simulink model "RequirementTable_testing"  (R2022b)
settings: Solver=FixedStepAuto  StartTime=0.0  StopTime=10.0  FixedStep=1e-3  RelTol=1e-3  EnableMultiTasking=on
undefined symbols (not defined in the file): D0, D1, D10, D11, D12, D13, D2, D3, D4, D5, D6, D7, D8, D9, PTA0, PTA1, PTA2, PTB23, PTB9, PTC16, PTC17, PTC2, PTC3, PTC4, PTD0, PTD1, PTD2, PTD3
libraries: frdmk64flib x18, dspstat3 x1
settings Model: SimulationMode=external  ExtModeTrigDuration=5  Creator=sarahalabdulrazzak  LastModifiedBy=coler
settings SolverCC: AlgebraicLoopSolver=TrustRegion
settings OptimizationCC: EnhancedBackFolding=on  PassReuseOutputArgsAs=Individual arguments  ZeroExternalMemoryAtStartup=off  ZeroInternalMemoryAtStartup=off  MaxStackSize=64  OptimizeBlockOrder=speed  DifferentSizesBufferReuse=on  OptimizationCustomize=off  EfficientTunableParamExpr=on
settings DebuggingCC: ParameterTunabilityLossMsg=error  UnconnectedInputMsg=warning  UnconnectedOutputMsg=warning  UnconnectedLineMsg=warning  SFMachineParentedDataDiag=warning
settings HardwareCC: ProdBitPerPointer=32  ProdBitPerSizeT=32  ProdBitPerPtrDiffT=32  ProdLargestAtomicInteger=Long  ProdLargestAtomicFloat=Double  ProdWordSize=32  ProdHWDeviceType=ARM Compatible->ARM Cortex
settings ModelReferenceCC: EnableRefExpFcnMdlSchedulingChecks=on
settings SFSimCC: MATLABDynamicMemAlloc=off
settings RTWCC: Description=Embedded Coder  SystemTargetFile=ert.tlc  HardwareBoard=NXP FRDM-K64F  TLCOptions="-aInlineSetEventsForThisBaseRateFcn=TLC_FALSE -aSuppressMultiTaskScheduler=TLC_FALSE  -aRateBasedStepFcn=0"  TemplateMakefile=ert_default_tmf  Toolchain=GNU Tools for ARM Embedded Processors
settings CodeAppCC: ForceParamTrailComments=on  IgnoreCustomStorageClasses=off  OperatorAnnotations=on  SimulinkDataObjDesc=on  SFDataObjDesc=on  InsertBlockDesc=on
settings ERTTargetCC: ExtMode=on  ExtModeTransport=4  ExtModeMexFile=sendToCommService  ExtModeMexArgs='RA_Modes' 0

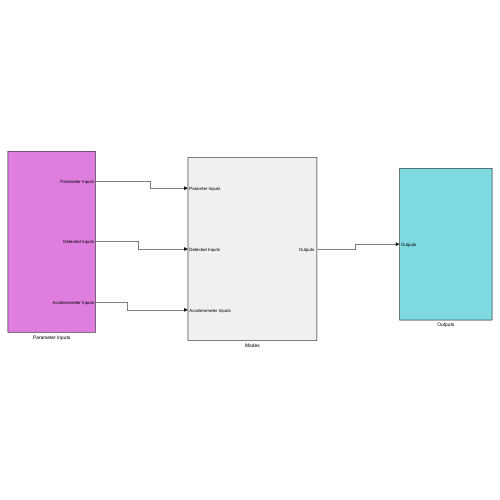
[thumbnail: Simulink's stored preview of the top-level diagram]
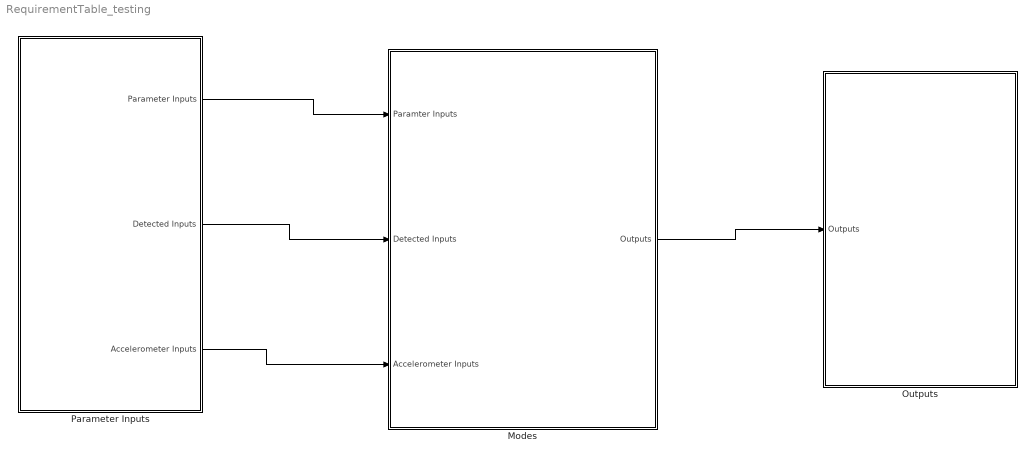
== system RequirementTable_testing ==
  Modes : Subsystem
  Outputs : Subsystem
  Parameter Inputs : Subsystem
  wires:
  Parameter Inputs/1(Parameter Inputs) -> Modes/1(Paramter Inputs)
  Parameter Inputs/2(Detected Inputs) -> Modes/2(Detected Inputs)
  Modes/1("Outputs ") -> Outputs/1("Outputs ")
  Parameter Inputs/3(Accelerometer Inputs) -> Modes/3(Accelerometer Inputs)

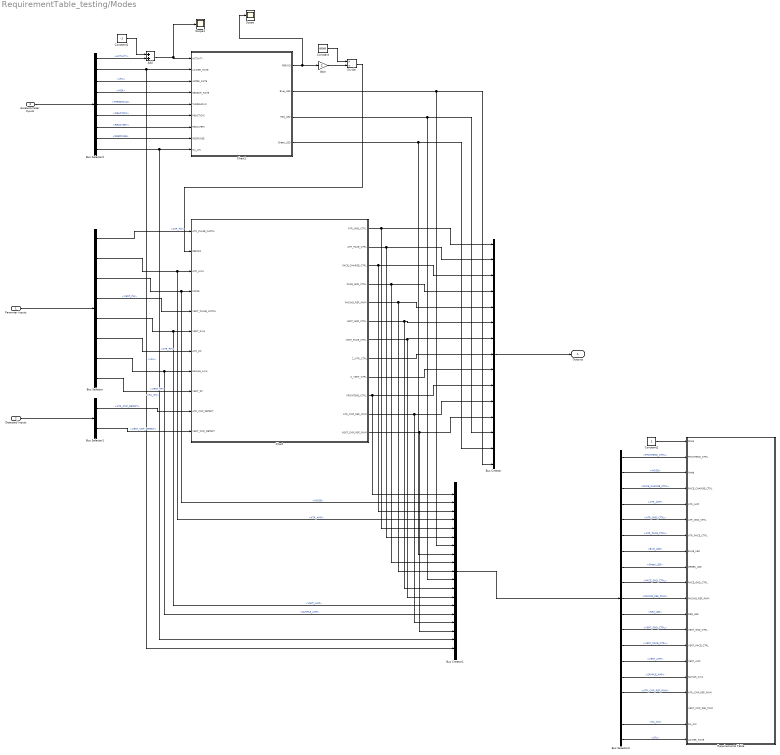
== system RequirementTable_testing/Modes ==
  Paramter Inputs : Inport
  Detected Inputs : Inport  Port=2
  Accelerometer Inputs : Inport  Port=3
  Add : Sum
  Bus Creator : BusCreator  Inputs=15
  Bus Creator1 : BusCreator  Inputs=19
  Bus Selector : BusSelector  OutputSignals=ATR_PW,ATR_AMP,MODE,VENT_PW,VENT_AMP,ATR_RP,SAMPLE_AMP,VENT_RP
  Bus Selector1 : BusSelector  OutputSignals=ATR_CMP_DETECT,VENT_CMP_DETECT
  Bus Selector2 : BusSelector  OutputSignals=ACTIVITY,LRL,URL,MSR,THRESHOLD,REACTION,RECOVERY,RESPONSE,RA_ON
  Bus Selector3 : BusSelector  OutputSignals=FRONTEND_CTRL,MODE,PACE_CHARGE_CTRL,ATR_AMP,ATR_GND_CTRL,ATR_PACE_CTRL,Blue_LED,Green_LED,PACE_GND_CTRL,PACING_REF_PWM,Red_LED,VENT_GND_CTRL,VENT_PACE_CTRL,VENT_AMP,SAMPLE_AMP,ATR_CMP_REF_PWM,VENT_CMP_REF_PWM,RA_ON,LRL
  Chart : Stateflow chart  TreatAsAtomicUnit=on
  Chart1 : Stateflow chart  TreatAsAtomicUnit=on
  Constant : Constant  Value=60000
  Constant1 : Constant  Value=-1
  Constant2 : Constant
  Divide : Product  Inputs=*/
  Gain : Gain  Gain=2
  Requirements Table : Requirements Table  TreatAsAtomicUnit=on
  Scope : Scope
  Scope1 : Scope
  "Outputs " : Outport
  wires:
  Paramter Inputs/1 -> Bus Selector/1
  Detected Inputs/1 -> Bus Selector1/1
  Bus Selector/1 -> Chart/1(ATR_PULSE_WIDTH)  "<ATR_PW>"
  Chart/1(ATR_GND_CTRL) -> Bus Creator1/5, Bus Creator/1
  Chart/2(ATR_PACE_CTRL) -> Bus Creator1/6, Bus Creator/2
  Chart/4(PACE_GND_CTRL) -> Bus Creator1/9, Bus Creator/4
  Chart/5(PACING_REF_PWM) -> Bus Creator1/10, Bus Creator/5
  Chart/6(VENT_GND_CTRL) -> Bus Creator1/12, Bus Creator/6
  Chart/7(VENT_PACE_CTRL) -> Bus Creator1/13, Bus Creator/7
  Chart/8(Z_ATR_CTRL) -> Bus Creator/8
  Chart/9(Z_VENT_CTRL) -> Bus Creator/9
  Chart/10(FRONTEND_CTRL) -> Bus Creator1/1, Bus Creator/10
  Chart/11(ATR_CMP_REF_PWM) -> Bus Creator1/16, Bus Creator/11
  Chart/12(VENT_CMP_REF_PWM) -> Bus Creator1/17, Bus Creator/12
  Bus Creator/1 -> "Outputs "/1
  Bus Selector1/1 -> Chart/10(ATR_CMP_DETECT)  "<ATR_CMP_DETECT>"
  Bus Selector1/2 -> Chart/11(VENT_CMP_DETECT)  "<VENT_CMP_DETECT>"
  Chart/3(PACE_CHARGE_CTRL) -> Bus Creator1/3, Bus Creator/3
  Bus Selector/2 -> Bus Creator1/4, Chart/3(ATR_Amp)  "<ATR_AMP>"
  Bus Selector/3 -> Bus Creator1/2, Chart/4(MODE)  "<MODE>"
  Bus Selector/4 -> Chart/5(VENT_PULSE_WIDTH)  "<VENT_PW>"
  Bus Selector/5 -> Bus Creator1/14, Chart/6(VENT_Amp)  "<VENT_AMP>"
  Bus Selector/6 -> Chart/7(ATR_RP)  "<ATR_RP>"
  Bus Selector/7 -> Bus Creator1/15, Chart/8(Sample_Amp)  "<SAMPLE_AMP>"
  Bus Selector/8 -> Chart/9(VENT_RP)  "<VENT_RP>"
  Accelerometer Inputs/1 -> Bus Selector2/1
  Bus Selector2/2 -> Bus Creator1/19, Chart1/2(LOWER_RATE)  "<LRL>"
  Bus Selector2/3 -> Chart1/3(UPPER_RATE)  "<URL>"
  Bus Selector2/4 -> Chart1/4(SENSOR_RATE)  "<MSR>"
  Bus Selector2/7 -> Chart1/7(RECOVERY)  "<RECOVERY>"
  Bus Selector2/8 -> Chart1/8(RESPONSE)  "<RESPONSE>"
  Bus Selector2/9 -> Bus Creator1/18, Chart1/9(RA_ON)  "<RA_ON>"
  Chart1/1(PERIOD) -> Scope/1, Gain/1
  Chart1/2(Blue_LED) -> Bus Creator1/7, Bus Creator/15
  Chart1/3(Red_LED) -> Bus Creator1/11, Bus Creator/13
  Chart1/4(Green_LED) -> Bus Creator1/8, Bus Creator/14
  Constant/1 -> Divide/1
  Divide/1 -> Chart/2(PERIOD)
  Gain/1 -> Divide/2
  Bus Selector2/5 -> Chart1/5(THRESHOLD)  "<THRESHOLD>"
  Bus Selector2/6 -> Chart1/6(REACTION)  "<REACTION>"
  Bus Selector2/1 -> Add/2  "<ACTIVITY>"
  Add/1 -> Scope1/1, Chart1/1(ACTIVITY)
  Constant1/1 -> Add/1
  Bus Creator1/1 -> Bus Selector3/1
  Bus Selector3/1 -> Requirements Table/2(FRONTEND_CTRL)  "<FRONTEND_CTRL>"
  Bus Selector3/2 -> Requirements Table/3(Mode)  "<MODE>"
  Bus Selector3/3 -> Requirements Table/4(PACE_CHARGE_CTRL)  "<PACE_CHARGE_CTRL>"
  Bus Selector3/4 -> Requirements Table/5(ATR_AMP)  "<ATR_AMP>"
  Bus Selector3/5 -> Requirements Table/6(ATR_GND_CTRL)  "<ATR_GND_CTRL>"
  Bus Selector3/6 -> Requirements Table/7(ATR_PACE_CTRL)  "<ATR_PACE_CTRL>"
  Bus Selector3/7 -> Requirements Table/8(BLUE_LED)  "<Blue_LED>"
  Bus Selector3/8 -> Requirements Table/9(GREEN_LED)  "<Green_LED>"
  Bus Selector3/9 -> Requirements Table/10(PACE_GND_CTRL)  "<PACE_GND_CTRL>"
  Bus Selector3/10 -> Requirements Table/11(PACING_REF_PWM)  "<PACING_REF_PWM>"
  Bus Selector3/11 -> Requirements Table/12(RED_LED)  "<Red_LED>"
  Bus Selector3/12 -> Requirements Table/13(VENT_GND_CTRL)  "<VENT_GND_CTRL>"
  Bus Selector3/13 -> Requirements Table/14(VENT_PACE_CTRL)  "<VENT_PACE_CTRL>"
  Bus Selector3/14 -> Requirements Table/15(VENT_AMP)  "<VENT_AMP>"
  Bus Selector3/15 -> Requirements Table/16(Sample_Amp)  "<SAMPLE_AMP>"
  Bus Selector3/16 -> Requirements Table/17(ATR_CMP_REF_PWM)  "<ATR_CMP_REF_PWM>"
  Bus Selector3/18 -> Requirements Table/19(RA_ON)  "<RA_ON>"
  Bus Selector3/19 -> Requirements Table/20(LOWER_RATE)  "<LRL>"
  Constant2/1 -> Requirements Table/1(State)

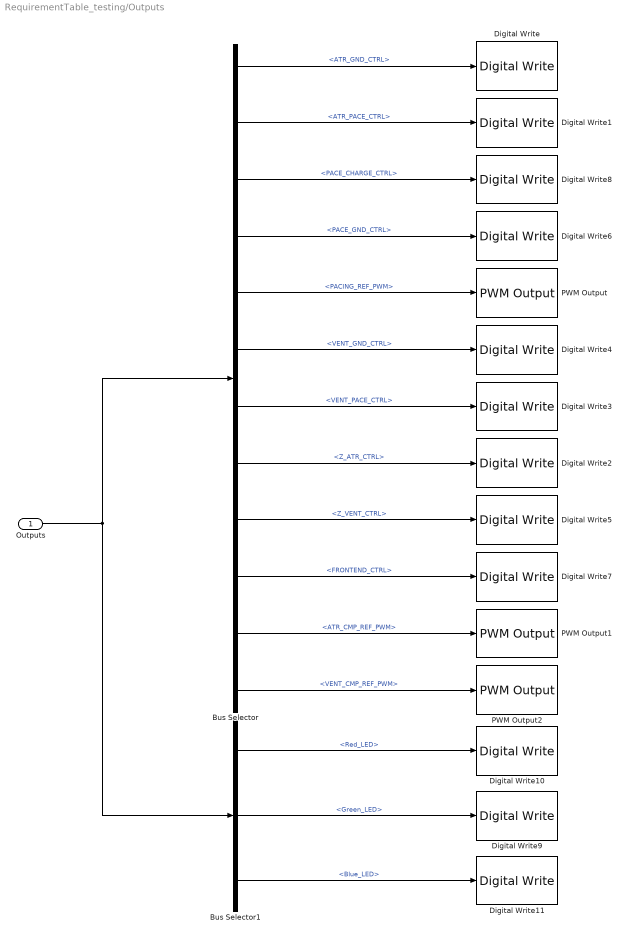
== system RequirementTable_testing/Outputs ==
  "Outputs " : Inport
  Bus Selector : BusSelector  OutputSignals=ATR_GND_CTRL,ATR_PACE_CTRL,PACE_CHARGE_CTRL,PACE_GND_CTRL,PACING_REF_PWM,VENT_GND_CTRL,VENT_PACE_CTRL,Z_ATR_CTRL,Z_VENT_CTRL,FRONTEND_CTRL,ATR_CMP_REF_PWM,VENT_CMP_REF_PWM
  Bus Selector1 : BusSelector  OutputSignals=Red_LED,Green_LED,Blue_LED
  Digital Write : frdmk64flib/Digital Write  Whichpin=PTD2 (D11)
  Digital Write1 : frdmk64flib/Digital Write  Whichpin=PTA0 (D8)
  Digital Write10 : frdmk64flib/Digital Write  Whichpin=RED_LED
  Digital Write11 : frdmk64flib/Digital Write  Whichpin=BLUE_LED
  Digital Write2 : frdmk64flib/Digital Write  Whichpin=PTB23 (D4)
  Digital Write3 : frdmk64flib/Digital Write  Whichpin=PTC4 (D9)
  Digital Write4 : frdmk64flib/Digital Write  Whichpin=PTD3 (D12)
  Digital Write5 : frdmk64flib/Digital Write  Whichpin=PTC3 (D7)
  Digital Write6 : frdmk64flib/Digital Write  Whichpin=PTD0 (D10)
  Digital Write7 : frdmk64flib/Digital Write  Whichpin=PTD1 (D13)
  Digital Write8 : frdmk64flib/Digital Write  Whichpin=PTB9 (D2)
  Digital Write9 : frdmk64flib/Digital Write  Whichpin=GREEN_LED
  PWM Output : frdmk64flib/PWM Output  Whichpin=PTA2 (D5)  InitialFrequency=2000  InitialDutyCycle=0
  PWM Output1 : frdmk64flib/PWM Output  Whichpin=PTC2 (D6)  InitialFrequency=2000  InitialDutyCycle=0
  PWM Output2 : frdmk64flib/PWM Output  Whichpin=PTA1 (D3)  InitialFrequency=2000  InitialDutyCycle=0
  wires:
  Bus Selector/1 -> Digital Write/1  "<ATR_GND_CTRL>"
  Bus Selector/2 -> Digital Write1/1  "<ATR_PACE_CTRL>"
  Bus Selector/3 -> Digital Write8/1  "<PACE_CHARGE_CTRL>"
  Bus Selector/4 -> Digital Write6/1  "<PACE_GND_CTRL>"
  Bus Selector/5 -> PWM Output/1  "<PACING_REF_PWM>"
  Bus Selector/6 -> Digital Write4/1  "<VENT_GND_CTRL>"
  Bus Selector/7 -> Digital Write3/1  "<VENT_PACE_CTRL>"
  Bus Selector/8 -> Digital Write2/1  "<Z_ATR_CTRL>"
  Bus Selector/9 -> Digital Write5/1  "<Z_VENT_CTRL>"
  Bus Selector/10 -> Digital Write7/1  "<FRONTEND_CTRL>"
  Bus Selector/11 -> PWM Output1/1  "<ATR_CMP_REF_PWM>"
  Bus Selector/12 -> PWM Output2/1  "<VENT_CMP_REF_PWM>"
  "Outputs "/1 -> Bus Selector/1, Bus Selector1/1
  Bus Selector1/1 -> Digital Write10/1  "<Red_LED>"
  Bus Selector1/2 -> Digital Write9/1  "<Green_LED>"
  Bus Selector1/3 -> Digital Write11/1  "<Blue_LED>"

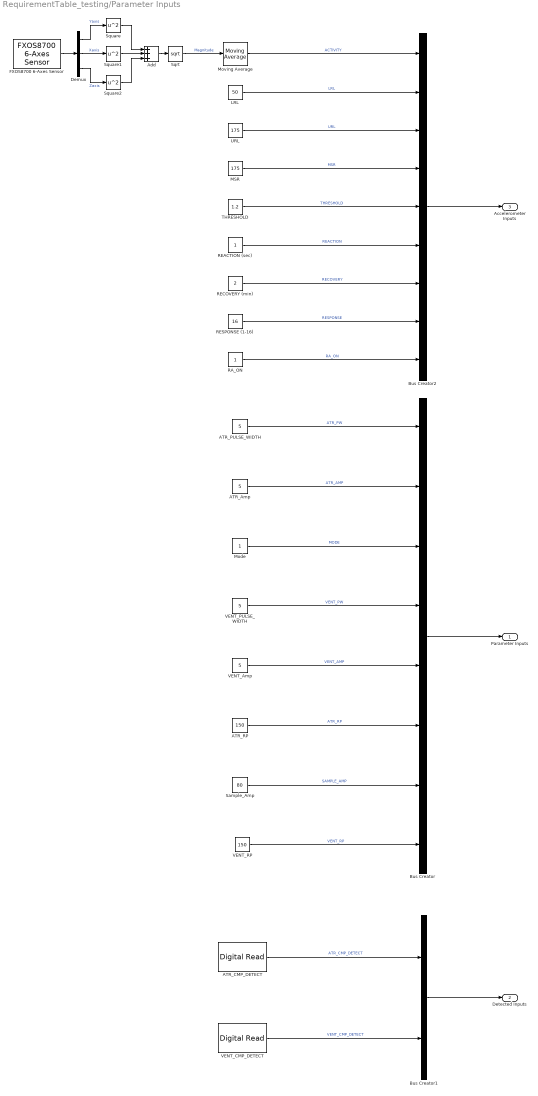
== system RequirementTable_testing/Parameter Inputs ==
  ATR_Amp : Constant  Value=5
  ATR_CMP_DETECT : frdmk64flib/Digital Read  Whichpin=PTC16 (D0)  SampleTime=-1
  ATR_PULSE_WIDTH : Constant  Value=5
  ATR_RP : Constant  Value=150
  Add : Sum  Inputs=+++
  Bus Creator : BusCreator  Inputs=8
  Bus Creator1 : BusCreator  Inputs=2
  Bus Creator2 : BusCreator  Inputs=9
  Demux : Demux  Outputs=3
  FXOS8700 6-Axes Sensor : frdmk64flib/FXOS8700 6-Axes Sensor  Activesensor=Accelerometer only  ODR=800Hz  HybridODR=400Hz  Accelfullrange=-4g to +4g  SampleTime=-1
  LRL : Constant  Value=50  OutDataTypeStr=double
  MSR : Constant  Value=175  OutDataTypeStr=double
  Mode : Constant
  Moving Average : dspstat3/Moving Average  Method=Exponential weighting  ForgettingFactorPort=off  SpecifyWindowLength=on  WindowLength=4  OverlapLength=3  AllowArbitraryInputLength=off  ForgettingFactor=0.999  SimulateUsing=Code generation
  RA_ON : Constant  OutDataTypeStr=boolean
  REACTION (sec) : Constant  OutDataTypeStr=double
  RECOVERY (min) : Constant  Value=2  OutDataTypeStr=double
  RESPONSE (1-16) : Constant  Value=16  OutDataTypeStr=double
  Sample_Amp : Constant  Value=80
  Sqrt : Sqrt
  Square : Math  Operator=square
  Square1 : Math  Operator=square
  Square2 : Math  Operator=square
  THRESHOLD : Constant  Value=1.2  OutDataTypeStr=double
  URL : Constant  Value=175  OutDataTypeStr=double
  VENT_Amp : Constant  Value=5
  VENT_CMP_DETECT : frdmk64flib/Digital Read  Whichpin=PTC17 (D1)  SampleTime=-1
  VENT_PULSE_WIDTH : Constant  Value=5
  VENT_RP : Constant  Value=150
  Parameter Inputs : Outport
  Detected Inputs : Outport  Port=2
  Accelerometer Inputs : Outport  Port=3
  wires:
  Bus Creator/1 -> Parameter Inputs/1
  ATR_PULSE_WIDTH/1 -> Bus Creator/1  "ATR_PW"
  ATR_Amp/1 -> Bus Creator/2  "ATR_AMP"
  Mode/1 -> Bus Creator/3  "MODE"
  VENT_PULSE_WIDTH/1 -> Bus Creator/4  "VENT_PW"
  VENT_Amp/1 -> Bus Creator/5  "VENT_AMP"
  ATR_RP/1 -> Bus Creator/6  "ATR_RP"
  Sample_Amp/1 -> Bus Creator/7  "SAMPLE_AMP"
  VENT_RP/1 -> Bus Creator/8  "VENT_RP"
  Bus Creator1/1 -> Detected Inputs/1
  VENT_CMP_DETECT/1 -> Bus Creator1/2  "VENT_CMP_DETECT"
  ATR_CMP_DETECT/1 -> Bus Creator1/1  "ATR_CMP_DETECT"
  Sqrt/1 -> Moving Average/1  "Magnitude"
  Demux/3 -> Square2/1  "Zaxis"
  Square2/1 -> Add/3
  Add/1 -> Sqrt/1
  Demux/2 -> Square1/1  "Xaxis"
  Square/1 -> Add/1
  Demux/1 -> Square/1  "Yaxis"
  FXOS8700 6-Axes Sensor/1 -> Demux/1
  Square1/1 -> Add/2
  Bus Creator2/1 -> Accelerometer Inputs/1
  Moving Average/1 -> Bus Creator2/1  "ACTIVITY"
  LRL/1 -> Bus Creator2/2  "LRL"
  URL/1 -> Bus Creator2/3  "URL"
  MSR/1 -> Bus Creator2/4  "MSR"
  RA_ON/1 -> Bus Creator2/9  "RA_ON"
  REACTION (sec)/1 -> Bus Creator2/6  "REACTION"
  THRESHOLD/1 -> Bus Creator2/5  "THRESHOLD"
  RECOVERY (min)/1 -> Bus Creator2/7  "RECOVERY"
  RESPONSE (1-16)/1 -> Bus Creator2/8  "RESPONSE"

== stateflow chart RequirementTable_testing/Modes/Chart1 ==
  state RECOVER_RATE
    %this is for if the RA is turned off while the
    %slowly shift activity (might not need)
    %if the period is above LRL, reduce by amount that will bring diff to 0 within recovery time
    Green_LED = true
    AVG_ACT = ACTIVITY
    if PERIOD > LOWER_RATE
    PERIOD = PERIOD - (SENSOR_RATE-LOWER_RATE)/(RECOVERY*1000)
    DELAY = (RECOVERY*1000)
    else
    PERIOD = LOWER_RATE
    DELAY = 0
    end
  state RA_OFF
    %set the period to LRL
    %read current activity
    %and assign to var.
    entry:
    PERIOD = LOWER_RATE
    AVG_ACT = ACTIVITY
    TH = single(THRESHOLD)
  state SET_TARGET
    %set the target rate and make sure it falls within the bounds
    Green_LED = false
    Red_LED = true
    TARGET_RATE = RESPONSE*((SENSOR_RATE - LOWER_RATE)/10)*ACTIVITY + LOWER_RATE
    %TARGET_RATE = 120
    if TARGET_RATE > SENSOR_RATE
    TARGET_RATE = SENSOR_RATE
    elseif TARGET_RATE < LOWER_RATE
    TARGET_RATE = LOWER_RATE
    end
  state RA_ON
    entry:
    Blue_LED = false
    Green_LED = false
    %Red_LED = false
  state RECOVER_REACT
    %slowly shift activity (might not need)
    %if Period is above target, decrease using recovery
    %if below target, increase using reaction
    Blue_LED = true
    AVG_ACT = ACTIVITY
    if PERIOD > TARGET_RATE
    PERIOD = PERIOD - (SENSOR_RATE-LOWER_RATE)/(RECOVERY*1000)
    DELAY = (RECOVERY*1000)
    elseif PERIOD < TARGET_RATE
    PERIOD = PERIOD + (SENSOR_RATE-LOWER_RATE)/(REACTION*1000)
    DELAY = (REACTION*1000)
    end
  RECOVER_RATE -> SET_TARGET [order 1] : [n >= DELAY && AVG_ACT >= TH]
  RECOVER_RATE -> RECOVER_RATE [order 2] : after(1,msec){n = n+1}
  RECOVER_RATE -> RA_OFF [order 3] : [RA_ON == FALSE && n >= DELAY]
  RA_ON -> RECOVER_RATE [order 1] : [AVG_ACT < TH]{n=0}
  (default) -> RA_OFF
  RA_ON -> SET_TARGET [order 2] : [AVG_ACT >= TH]
  RA_OFF -> RA_ON : [RA_ON == TRUE]{TARGET_RATE=PERIOD}
  RECOVER_REACT -> RA_ON [order 1] : [n >= DELAY]
  SET_TARGET -> RECOVER_REACT : {n=0, AVG_ACT = ACTIVITY}
  RECOVER_REACT -> RECOVER_REACT [order 2] : after(1,msec){n = n+1}
  data: ACTIVITY input; LOWER_RATE input; UPPER_RATE input; SENSOR_RATE input; THRESHOLD input; REACTION input; RECOVERY input; RESPONSE input; RA_ON input; PERIOD output double; TRUE local =1; FALSE local =0; TARGET_RATE local double; DELAY local double; n local; Blue_LED output; Red_LED output; Green_LED output; TH local; AVG_ACT local

== stateflow chart RequirementTable_testing/Modes/Requirements Table ==
  (default) -> (junction 1073745773)
  (junction 1073745773) -> (junction 1073745774) : {
      | % SF_REQ_REV_07
      | }
  (junction 1073745774) -> (junction 1073745776) : {
      | % HEADER_ASSIGNMENTS
      |
      | }
  (junction 1073745776) -> (junction 1073745778) : {
      | % START_A_4
      | }
  (junction 1073745778) -> (junction 1073745780) : {
      | }
  (junction 1073745780) -> (junction 1073745782) : {
      | reqtable_assumption(([0,3]), 4);
      | }
  (junction 1073745782) -> (junction 1073745784) : {
      | }
  (junction 1073745784) -> (junction 1073745786) : {
      | % END_A_4
      | }
  (junction 1073745786) -> (junction 1073745788) : {
      | % START_A_28
      | }
  (junction 1073745788) -> (junction 1073745790) : {
      | }
  (junction 1073745790) -> (junction 1073745792) : {
      | reqtable_assumption(([0,1]), 28);
      | }
  (junction 1073745792) -> (junction 1073745794) : {
      | }
  (junction 1073745794) -> (junction 1073745796) : {
      | % END_A_28
      | }
  (junction 1073745796) -> (junction 1073745798) : {
      | % START_R_1
      | }
  (junction 1073745798) -> (junction 1073745800) : {
      | }
  (junction 1073745800) -> (junction 1073745802)
  (junction 1073745802) -> (junction 1073745804) [order 1] : [(((RA_ON) == (0))) && (((Mode) == (1))) && (((State) == (0)))]
  (junction 1073745802) -> (junction 1073745810) [order 2]
  (junction 1073745804) -> (junction 1073745806) : {
      | reqtable_postcondition((((PACE_CHARGE_CTRL) == (1))) && (ATR_PACE_CTRL == 0) && (((PACING_REF_PWM ) == (ATR_AMP))) && (((PACE_CHARGE_CTRL) == (1))) && (((PACE_GND_CTRL) == (1))) && (ATR_GND_CTRL == 1) && (((RED_LED) == (0))) && (((GREEN_LED) == (0))) && (((BLUE_LED) == (0))) && (abs(time-get_param('SimulationTime')) / (60*1000) >= LOWER_RATE), 'R:1');
      |
      | }
  (junction 1073745806) -> (junction 1073745808) : {
      | }
  (junction 1073745808) -> (junction 1073745810)
  (junction 1073745810) -> (junction 1073745812)
  (junction 1073745812) -> (junction 1073745814) : {
      | % END_R_1
      | }
  (junction 1073745814) -> (junction 1073745816) : {
      | % START_R_82
      | }
  (junction 1073745816) -> (junction 1073745818) : {
      | }
  (junction 1073745818) -> (junction 1073745820)
  (junction 1073745820) -> (junction 1073745822) [order 1] : [(((RA_ON) == (1))) && (((Mode) == (1))) && (((State) == (0)))]
  (junction 1073745820) -> (junction 1073745828) [order 2]
  (junction 1073745822) -> (junction 1073745824) : {
      | reqtable_postcondition((((PACE_CHARGE_CTRL) == (1))) && (ATR_PACE_CTRL == 0) && (((PACING_REF_PWM ) == (ATR_AMP))) && (((PACE_CHARGE_CTRL) == (1))) && (((PACE_GND_CTRL) == (1))) && (ATR_GND_CTRL == 1) && (((RED_LED) == (0))) && (((GREEN_LED) == (0))) && (((BLUE_LED) == (0))) && (abs(time-get_param('SimulationTime')) / (60*1000) >= TARGET_RATE-5), 'R:2');
      |
      | }
  (junction 1073745824) -> (junction 1073745826) : {
      | }
  (junction 1073745826) -> (junction 1073745828)
  (junction 1073745828) -> (junction 1073745830)
  (junction 1073745830) -> (junction 1073745832) : {
      | % END_R_82
      | }
  (junction 1073745832) -> (junction 1073745834) : {
      | % START_R_7
      | }
  (junction 1073745834) -> (junction 1073745836) : {
      | }
  (junction 1073745836) -> (junction 1073745838)
  (junction 1073745838) -> (junction 1073745840) [order 1] : [(((RA_ON) == (0))) && (((Mode) == (1))) && (((State) == (1)))]
  (junction 1073745838) -> (junction 1073745846) [order 2]
  (junction 1073745840) -> (junction 1073745842) : {
      | reqtable_postcondition((((PACE_CHARGE_CTRL) == (0))) && (ATR_PACE_CTRL == 1) && (((PACING_REF_PWM ) == (ATR_AMP))) && (((PACE_CHARGE_CTRL) == (0))) && (((PACE_GND_CTRL) == (1))) && (ATR_GND_CTRL == 0) && (((RED_LED) == (1))) && (((GREEN_LED) == (0))) && (((BLUE_LED) == (0))) && (abs(time-get_param('SimulationTime')) / (60*1000) >= LOWER_RATE), 'R:3');
      |
      | }
  (junction 1073745842) -> (junction 1073745844) : {
      | }
  (junction 1073745844) -> (junction 1073745846)
  (junction 1073745846) -> (junction 1073745848)
  (junction 1073745848) -> (junction 1073745850) : {
      | % END_R_7
      | }
  (junction 1073745850) -> (junction 1073745852) : {
      | % START_R_88
      | }
  (junction 1073745852) -> (junction 1073745854) : {
      | }
  (junction 1073745854) -> (junction 1073745856)
  (junction 1073745856) -> (junction 1073745858) [order 1] : [(((RA_ON) == (1))) && (((Mode) == (1))) && (((State) == (1)))]
  (junction 1073745856) -> (junction 1073745864) [order 2]
  (junction 1073745858) -> (junction 1073745860) : {
      | reqtable_postcondition((((PACE_CHARGE_CTRL) == (0))) && (ATR_PACE_CTRL == 1) && (((PACING_REF_PWM ) == (ATR_AMP))) && (((PACE_CHARGE_CTRL) == (0))) && (((PACE_GND_CTRL) == (1))) && (ATR_GND_CTRL == 0) && (((RED_LED) == (1))) && (((GREEN_LED) == (0))) && (((BLUE_LED) == (0))) && (abs(time-get_param('SimulationTime')) / (60*1000) >= TARGET_RATE-5), 'R:4');
      |
      | }
  (junction 1073745860) -> (junction 1073745862) : {
      | }
  (junction 1073745862) -> (junction 1073745864)
  (junction 1073745864) -> (junction 1073745866)
  (junction 1073745866) -> (junction 1073745868) : {
      | % END_R_88
      | }
  (junction 1073745868) -> (junction 1073745870) : {
      | % START_R_10
      | }
  (junction 1073745870) -> (junction 1073745872) : {
      | }
  (junction 1073745872) -> (junction 1073745874)
  (junction 1073745874) -> (junction 1073745876) [order 1] : [(((RA_ON) == (0))) && (((Mode) == (3))) && (((State) == (0)))]
  (junction 1073745874) -> (junction 1073745882) [order 2]
  (junction 1073745876) -> (junction 1073745878) : {
      | reqtable_postcondition((((PACE_CHARGE_CTRL) == (1))) && (VENT_PACE_CTRL == 0) && (((PACING_REF_PWM ) == (VENT_AMP))) && (((PACE_CHARGE_CTRL) == (1))) && (((PACE_GND_CTRL) == (1))) && (VENT_GND_CTRL == 1) && (((RED_LED) == (0))) && (((GREEN_LED) == (0))) && (((BLUE_LED) == (0))) && (abs(time-get_param('SimulationTime')) / (60*1000) >= LOWER_RATE), 'R:5');
      |
      | }
  (junction 1073745878) -> (junction 1073745880) : {
      | }
  (junction 1073745880) -> (junction 1073745882)
  (junction 1073745882) -> (junction 1073745884)
  (junction 1073745884) -> (junction 1073745886) : {
      | % END_R_10
      | }
  (junction 1073745886) -> (junction 1073745888) : {
      | % START_R_85
      | }
  (junction 1073745888) -> (junction 1073745890) : {
      | }
  (junction 1073745890) -> (junction 1073745892)
  (junction 1073745892) -> (junction 1073745894) [order 1] : [(((RA_ON) == (1))) && (((Mode) == (3))) && (((State) == (0)))]
  (junction 1073745892) -> (junction 1073745900) [order 2]
  (junction 1073745894) -> (junction 1073745896) : {
      | reqtable_postcondition((((PACE_CHARGE_CTRL) == (1))) && (VENT_PACE_CTRL == 0) && (((PACING_REF_PWM ) == (VENT_AMP))) && (((PACE_CHARGE_CTRL) == (1))) && (((PACE_GND_CTRL) == (1))) && (VENT_GND_CTRL == 1) && (((RED_LED) == (0))) && (((GREEN_LED) == (0))) && (((BLUE_LED) == (0))) && (abs(time-get_param('SimulationTime')) / (60*1000) >= TARGET_RATE-5), 'R:6');
      |
      | }
  (junction 1073745896) -> (junction 1073745898) : {
      | }
  (junction 1073745898) -> (junction 1073745900)
  (junction 1073745900) -> (junction 1073745902)
  (junction 1073745902) -> (junction 1073745904) : {
      | % END_R_85
      | }
  (junction 1073745904) -> (junction 1073745906) : {
      | % START_R_13
      | }
  (junction 1073745906) -> (junction 1073745908) : {
      | }
  (junction 1073745908) -> (junction 1073745910)
  (junction 1073745910) -> (junction 1073745912) [order 1] : [(((RA_ON) == (0))) && (((Mode) == (3))) && (((State) == (1)))]
  (junction 1073745910) -> (junction 1073745918) [order 2]
  (junction 1073745912) -> (junction 1073745914) : {
      | reqtable_postcondition((((PACE_CHARGE_CTRL) == (0))) && (VENT_PACE_CTRL == 1) && (((PACING_REF_PWM ) == (VENT_AMP))) && (((PACE_CHARGE_CTRL) == (0))) && (((PACE_GND_CTRL) == (1))) && (VENT_GND_CTRL == 0) && (((RED_LED) == (0))) && (((GREEN_LED) == (1))) && (((BLUE_LED) == (0))) && (abs(time-get_param('SimulationTime')) / (60*1000) >= LOWER_RATE), 'R:7');
      |
      | }
  (junction 1073745914) -> (junction 1073745916) : {
      | }
  (junction 1073745916) -> (junction 1073745918)
  (junction 1073745918) -> (junction 1073745920)
  (junction 1073745920) -> (junction 1073745922) : {
      | % END_R_13
      | }
  (junction 1073745922) -> (junction 1073745924) : {
      | % START_R_91
      | }
  (junction 1073745924) -> (junction 1073745926) : {
      | }
  (junction 1073745926) -> (junction 1073745928)
  (junction 1073745928) -> (junction 1073745930) [order 1] : [(((RA_ON) == (1))) && (((Mode) == (3))) && (((State) == (1)))]
  (junction 1073745928) -> (junction 1073745936) [order 2]
  (junction 1073745930) -> (junction 1073745932) : {
      | reqtable_postcondition((((PACE_CHARGE_CTRL) == (0))) && (VENT_PACE_CTRL == 1) && (((PACING_REF_PWM ) == (VENT_AMP))) && (((PACE_CHARGE_CTRL) == (0))) && (((PACE_GND_CTRL) == (1))) && (VENT_GND_CTRL == 0) && (((RED_LED) == (0))) && (((GREEN_LED) == (1))) && (((BLUE_LED) == (0))) && (abs(time-get_param('SimulationTime')) / (60*1000) >= TARGET_RATE-5), 'R:8');
      |
      | }
  (junction 1073745932) -> (junction 1073745934) : {
      | }
  (junction 1073745934) -> (junction 1073745936)
  (junction 1073745936) -> (junction 1073745938)
  (junction 1073745938) -> (junction 1073745940) : {
      | % END_R_91
      | }
  (junction 1073745940) -> (junction 1073745942) : {
      | % START_R_16
      | }
  (junction 1073745942) -> (junction 1073745944) : {
      | }
  (junction 1073745944) -> (junction 1073745946)
  (junction 1073745946) -> (junction 1073745948) [order 1] : [(((RA_ON) == (0))) && (((Mode) == (2))) && (((State) == (0))) && (FRONTEND_CTRL == 1)]
  (junction 1073745946) -> (junction 1073745954) [order 2]
  (junction 1073745948) -> (junction 1073745950) : {
      | reqtable_postcondition((((PACE_CHARGE_CTRL) == (1))) && (ATR_PACE_CTRL == 0) && (((PACING_REF_PWM ) == (ATR_AMP))) && (((PACE_CHARGE_CTRL) == (1))) && (((PACE_GND_CTRL) == (1))) && (ATR_GND_CTRL == 1) && (((RED_LED) == (0))) && (((GREEN_LED) == (0))) && (((BLUE_LED) == (0))) && (ATR_CMP_REF_PWM == Sample_Amp) && (abs(time-get_param('SimulationTime')) / (60*1000) >= LOWER_RATE), 'R:9');
      |
      | }
  (junction 1073745950) -> (junction 1073745952) : {
      | }
  (junction 1073745952) -> (junction 1073745954)
  (junction 1073745954) -> (junction 1073745956)
  (junction 1073745956) -> (junction 1073745958) : {
      | % END_R_16
      | }
  (junction 1073745958) -> (junction 1073745960) : {
      | % START_R_94
      | }
  (junction 1073745960) -> (junction 1073745962) : {
      | }
  (junction 1073745962) -> (junction 1073745964)
  (junction 1073745964) -> (junction 1073745966) [order 1] : [(((RA_ON) == (1))) && (((Mode) == (2))) && (((State) == (0))) && (FRONTEND_CTRL == 1)]
  (junction 1073745964) -> (junction 1073745972) [order 2]
  (junction 1073745966) -> (junction 1073745968) : {
      | reqtable_postcondition((((PACE_CHARGE_CTRL) == (1))) && (ATR_PACE_CTRL == 0) && (((PACING_REF_PWM ) == (ATR_AMP))) && (((PACE_CHARGE_CTRL) == (1))) && (((PACE_GND_CTRL) == (1))) && (ATR_GND_CTRL == 1) && (((RED_LED) == (0))) && (((GREEN_LED) == (0))) && (((BLUE_LED) == (0))) && (ATR_CMP_REF_PWM == Sample_Amp) && (abs(time-get_param('SimulationTime')) / (60*1000) >= TARGET_RATE-5), 'R:10');
      |
      | }
  (junction 1073745968) -> (junction 1073745970) : {
      | }
  (junction 1073745970) -> (junction 1073745972)
  (junction 1073745972) -> (junction 1073745974)
  (junction 1073745974) -> (junction 1073745976) : {
      | % END_R_94
      | }
  (junction 1073745976) -> (junction 1073745978) : {
      | % START_R_19
      | }
  (junction 1073745978) -> (junction 1073745980) : {
      | }
  (junction 1073745980) -> (junction 1073745982)
  (junction 1073745982) -> (junction 1073745984) [order 1] : [(((RA_ON) == (0))) && (((Mode) == (2))) && (((State) == (1)))]
  (junction 1073745982) -> (junction 1073745990) [order 2]
  (junction 1073745984) -> (junction 1073745986) : {
      | reqtable_postcondition((((PACE_CHARGE_CTRL) == (0))) && (ATR_PACE_CTRL == 1) && (((PACING_REF_PWM ) == (ATR_AMP))) && (((PACE_CHARGE_CTRL) == (0))) && (((PACE_GND_CTRL) == (1))) && (ATR_GND_CTRL == 0) && (((RED_LED) == (0))) && (((GREEN_LED) == (0))) && (((BLUE_LED) == (0))) && (ATR_CMP_REF_PWM == Sample_Amp) && (abs(time-get_param('SimulationTime')) / (60*1000) >= LOWER_RATE), 'R:11');
      |
      | }
  (junction 1073745986) -> (junction 1073745988) : {
      | }
  (junction 1073745988) -> (junction 1073745990)
  (junction 1073745990) -> (junction 1073745992)
  (junction 1073745992) -> (junction 1073745994) : {
      | % END_R_19
      | }
  (junction 1073745994) -> (junction 1073745996) : {
      | % START_R_97
      | }
  (junction 1073745996) -> (junction 1073745998) : {
      | }
  (junction 1073745998) -> (junction 1073746000)
  (junction 1073746000) -> (junction 1073746002) [order 1] : [(((RA_ON) == (1))) && (((Mode) == (2))) && (((State) == (1)))]
  (junction 1073746000) -> (junction 1073746008) [order 2]
  (junction 1073746002) -> (junction 1073746004) : {
      | reqtable_postcondition((((PACE_CHARGE_CTRL) == (0))) && (ATR_PACE_CTRL == 1) && (((PACING_REF_PWM ) == (ATR_AMP))) && (((PACE_CHARGE_CTRL) == (0))) && (((PACE_GND_CTRL) == (1))) && (ATR_GND_CTRL == 0) && (((RED_LED) == (0))) && (((GREEN_LED) == (0))) && (((BLUE_LED) == (0))) && (ATR_CMP_REF_PWM == Sample_Amp) && (abs(time-get_param('SimulationTime')) / (60*1000) >= TARGET_RATE-5), 'R:12');
      |
      | }
  (junction 1073746004) -> (junction 1073746006) : {
      | }
  (junction 1073746006) -> (junction 1073746008)
  (junction 1073746008) -> (junction 1073746010)
  (junction 1073746010) -> (junction 1073746012) : {
      | % END_R_97
      | }
  (junction 1073746012) -> (junction 1073746014) : {
      | % START_R_22
      | }
  (junction 1073746014) -> (junction 1073746016) : {
      | }
  (junction 1073746016) -> (junction 1073746018)
  (junction 1073746018) -> (junction 1073746020) [order 1] : [(((RA_ON) == (0))) && (((Mode) == (4))) && (((State) == (0))) && (FRONTEND_CTRL == 1)]
  (junction 1073746018) -> (junction 1073746026) [order 2]
  (junction 1073746020) -> (junction 1073746022) : {
      | reqtable_postcondition((((PACE_CHARGE_CTRL) == (1))) && (VENT_PACE_CTRL == 0) && (((PACING_REF_PWM ) == (VENT_AMP))) && (((PACE_CHARGE_CTRL) == (1))) && (((PACE_GND_CTRL) == (1))) && (VENT_GND_CTRL == 1) && (((RED_LED) == (0))) && (((GREEN_LED) == (0))) && (((BLUE_LED) == (0))) && (VENT_CMP_REF_PWM == Sample_Amp) && (abs(time-get_param('SimulationTime')) / (60*1000) >= LOWER_RATE), 'R:13');
      |
      | }
  (junction 1073746022) -> (junction 1073746024) : {
      | }
  (junction 1073746024) -> (junction 1073746026)
  (junction 1073746026) -> (junction 1073746028)
  (junction 1073746028) -> (junction 1073746030) : {
      | % END_R_22
      | }
  (junction 1073746030) -> (junction 1073746032) : {
      | % START_R_100
      | }
  (junction 1073746032) -> (junction 1073746034) : {
      | }
  (junction 1073746034) -> (junction 1073746036)
  (junction 1073746036) -> (junction 1073746038) [order 1] : [(((RA_ON) == (1))) && (((Mode) == (4))) && (((State) == (0))) && (FRONTEND_CTRL == 1)]
  (junction 1073746036) -> (junction 1073746044) [order 2]
  (junction 1073746038) -> (junction 1073746040) : {
      | reqtable_postcondition((((PACE_CHARGE_CTRL) == (1))) && (VENT_PACE_CTRL == 0) && (((PACING_REF_PWM ) == (VENT_AMP))) && (((PACE_CHARGE_CTRL) == (1))) && (((PACE_GND_CTRL) == (1))) && (VENT_GND_CTRL == 1) && (((RED_LED) == (0))) && (((GREEN_LED) == (0))) && (((BLUE_LED) == (0))) && (VENT_CMP_REF_PWM == Sample_Amp) && (abs(time-get_param('SimulationTime')) / (60*1000) >= TARGET_RATE-5), 'R:14');
      |
      | }
  (junction 1073746040) -> (junction 1073746042) : {
      | }
  (junction 1073746042) -> (junction 1073746044)
  (junction 1073746044) -> (junction 1073746046)
  (junction 1073746046) -> (junction 1073746048) : {
      | % END_R_100
      | }
  (junction 1073746048) -> (junction 1073746050) : {
      | % START_R_25
      | }
  (junction 1073746050) -> (junction 1073746052) : {
      | }
  (junction 1073746052) -> (junction 1073746054)
  (junction 1073746054) -> (junction 1073746056) [order 1] : [(((RA_ON) == (0))) && (((Mode) == (4))) && (((State) == (1)))]
  (junction 1073746054) -> (junction 1073746062) [order 2]
  (junction 1073746056) -> (junction 1073746058) : {
      | reqtable_postcondition((((PACE_CHARGE_CTRL) == (0))) && (VENT_PACE_CTRL == 1) && (((PACING_REF_PWM ) == (VENT_AMP))) && (((PACE_CHARGE_CTRL) == (0))) && (((PACE_GND_CTRL) == (1))) && (VENT_GND_CTRL == 0) && (((RED_LED) == (0))) && (((GREEN_LED) == (1))) && (((BLUE_LED) == (0))) && (VENT_CMP_REF_PWM == Sample_Amp) && (abs(time-get_param('SimulationTime')) / (60*1000) >= LOWER_RATE), 'R:15');
      |
      | }
  (junction 1073746058) -> (junction 1073746060) : {
      | }
  (junction 1073746060) -> (junction 1073746062)
  (junction 1073746062) -> (junction 1073746064)
  (junction 1073746064) -> (junction 1073746066) : {
      | % END_R_25
      | }
  (junction 1073746066) -> (junction 1073746068) : {
      | % START_R_103
      | }
  (junction 1073746068) -> (junction 1073746070) : {
      | }
  (junction 1073746070) -> (junction 1073746072)
  (junction 1073746072) -> (junction 1073746074) [order 1] : [(((RA_ON) == (1))) && (((Mode) == (4))) && (((State) == (1)))]
  (junction 1073746072) -> (junction 1073746080) [order 2]
  (junction 1073746074) -> (junction 1073746076) : {
      | reqtable_postcondition((((PACE_CHARGE_CTRL) == (0))) && (VENT_PACE_CTRL == 1) && (((PACING_REF_PWM ) == (VENT_AMP))) && (((PACE_CHARGE_CTRL) == (0))) && (((PACE_GND_CTRL) == (1))) && (VENT_GND_CTRL == 0) && (((RED_LED) == (0))) && (((GREEN_LED) == (1))) && (((BLUE_LED) == (0))) && (VENT_CMP_REF_PWM == Sample_Amp) && (abs(time-get_param('SimulationTime')) / (60*1000) >= TARGET_RATE-5), 'R:16');
      |
      | }
  (junction 1073746076) -> (junction 1073746078) : {
      | }
  (junction 1073746078) -> (junction 1073746080)
  (junction 1073746080) -> (junction 1073746082)
  (junction 1073746082) -> (junction 1073746084) : {
      | % END_R_103
      | }
  data: State input; FRONTEND_CTRL input; Mode input; PACE_CHARGE_CTRL input; ATR_AMP input; ATR_GND_CTRL input; ATR_PACE_CTRL input; BLUE_LED input; GREEN_LED input; PACE_GND_CTRL input; PACING_REF_PWM input; RED_LED input; VENT_GND_CTRL input; VENT_PACE_CTRL input; VENT_AMP input; Sample_Amp input; ATR_CMP_REF_PWM input; VENT_CMP_REF_PWM input; time local; RA_ON input; LOWER_RATE input

== stateflow chart RequirementTable_testing/Modes/Chart ==
  state Identify_Mode_Path
    entry:
    % MODE = 1 (AOO)
    % MODE = 2 (AAI)
    % MODE = 3 (VOO)
    % MODE = 4 (VVI)
    %
    %pacemaker disconnected
    %stop sensing
    PACE_CHARGE_CTRL = LOW
    VENT_PACE_CTRL = LOW
    ATR_PACE_CTRL = LOW
    PACE_GND_CTRL = LOW
    ATR_GND_CTRL = LOW
    VENT_GND_CTRL = LOW
    Z_ATR_CTRL = LOW
    Z_VENT_CTRL = LOW
    FRONTEND_CTRL = LOW
  state AOO
    entry:
    %Charge primary capcitor C22
    ATR_PACE_CTRL=LOW
    PACING_REF_PWM = 20*ATR_Amp
    PACE_CHARGE_CTRL = HIGH
    %Discharge block capacitor C21
    PACE_GND_CTRL = HIGH
    ATR_GND_CTRL = HIGH
    %use LED  to verify state
  state AOO_ATR_PULSE
    entry:
    %Discharge C22 primary capacitor
    %Charge C21 block capacitor
    PACE_CHARGE_CTRL = LOW
    PACE_GND_CTRL = HIGH
    ATR_PACE_CTRL = HIGH
    ATR_GND_CTRL = LOW
    PACING_REF_PWM = 20*ATR_Amp
    %use LED  to verify state
  state AAI
    entry:
    %sensing ON
    FRONTEND_CTRL = HIGH
    %Charge primary capcitor C22
    ATR_PACE_CTRL=LOW
    PACING_REF_PWM = 20*ATR_Amp
    PACE_CHARGE_CTRL = HIGH
    %Discharge block capacitor C21
    PACE_GND_CTRL = HIGH
    ATR_GND_CTRL = HIGH
    ATR_CMP_REF_PWM = Sample_Amp
    %use LED  to verify state
  state AAI_ATR_PULSE
    entry:
    %sensing OFF
    FRONTEND_CTRL = LOW
    %Discharge C22 primary capacitor
    %Charge C21 block capacitor
    PACE_CHARGE_CTRL = LOW
    PACE_GND_CTRL = HIGH
    ATR_PACE_CTRL = HIGH
    ATR_GND_CTRL = LOW
    PACING_REF_PWM = 20*ATR_Amp
    %use LED  to verify state
  state VOO
    entry:
    %Charge primary capcitor C22
    VENT_PACE_CTRL=LOW
    PACING_REF_PWM = 20*VENT_Amp
    PACE_CHARGE_CTRL = HIGH
    %Discharge block capacitor C21
    PACE_GND_CTRL = HIGH
    VENT_GND_CTRL = HIGH
    %use LED  to verify state
  state VOO_VENT_PULSE
    entry:
    %Discharge C22 primary capacitor
    %Charge C21 block capacitor
    PACE_CHARGE_CTRL = LOW
    PACE_GND_CTRL = HIGH
    VENT_GND_CTRL = LOW
    VENT_PACE_CTRL  = HIGH
    PACING_REF_PWM = 20*VENT_Amp
    %use LED  to verify state
  state VVI
    entry:
    %sensing ON
    FRONTEND_CTRL = HIGH
    %Charge primary capcitor C22
    VENT_PACE_CTRL= LOW
    PACING_REF_PWM = 20*VENT_Amp
    PACE_CHARGE_CTRL = HIGH
    %Discharge block capacitor C21
    PACE_GND_CTRL = HIGH
    VENT_PACE_CTRL = LOW
    VENT_GND_CTRL = HIGH
    VENT_CMP_REF_PWM = Sample_Amp
    %use LED  to verify state
  state VVI_VENT_PULSE
    %sensing OFF
    FRONTEND_CTRL = LOW
    %Discharge C22 primary capacitor
    %Charge C21 block capacitor
    PACE_CHARGE_CTRL = LOW
    PACE_GND_CTRL = HIGH
    VENT_GND_CTRL = LOW
    VENT_PACE_CTRL  = HIGH
    PACING_REF_PWM = 20*VENT_Amp
    %use LED  to verify state
  (default) -> Identify_Mode_Path
  AOO -> AOO_ATR_PULSE [order 1] : after(PERIOD - ATR_PULSE_WIDTH,msec)
  Identify_Mode_Path -> AOO [order 1] : [MODE == 1]
  AOO_ATR_PULSE -> AOO : after(ATR_PULSE_WIDTH,msec)
  AOO -> Identify_Mode_Path [order 2] : [MODE ~= 1]
  AAI_ATR_PULSE -> AAI : after(ATR_PULSE_WIDTH,msec)
  Identify_Mode_Path -> AAI [order 2] : [MODE == 2]
  AAI -> (junction 41) [order 1]
  (junction 41) -> AAI_ATR_PULSE [order 1] : after(PERIOD - ATR_PULSE_WIDTH,msec)[ATR_CMP_DETECT == LOW]
  (junction 41) -> AAI [order 2] : after(ATR_RP, msec)[ATR_CMP_DETECT == HIGH]
  AAI -> Identify_Mode_Path [order 2] : [MODE ~= 2]
  VOO -> VOO_VENT_PULSE [order 1] : after(PERIOD - VENT_PULSE_WIDTH,msec)
  Identify_Mode_Path -> VOO [order 3] : [MODE == 3]
  VOO_VENT_PULSE -> VOO : after(VENT_PULSE_WIDTH,msec)
  VOO -> Identify_Mode_Path [order 2] : [MODE ~= 3]
  VVI_VENT_PULSE -> VVI : after(VENT_PULSE_WIDTH,msec)
  Identify_Mode_Path -> VVI [order 4] : [MODE == 4]
  VVI -> (junction 61) [order 1]
  (junction 61) -> VVI_VENT_PULSE [order 1] : after(PERIOD - VENT_PULSE_WIDTH,msec)[VENT_CMP_DETECT == LOW]
  (junction 61) -> VVI [order 2] : after(VENT_RP, msec)[VENT_CMP_DETECT == HIGH]
  VVI -> Identify_Mode_Path [order 2] : [MODE ~= 4]
  data: ATR_PULSE_WIDTH input; PERIOD input; ATR_Amp input; MODE input; VENT_PULSE_WIDTH input; VENT_Amp input; ATR_RP input; Sample_Amp input; VENT_RP input; ATR_CMP_DETECT input; VENT_CMP_DETECT input; HIGH local =1; LOW local =0; ATR_GND_CTRL output; ATR_PACE_CTRL output; PACE_CHARGE_CTRL output; PACE_GND_CTRL output; PACING_REF_PWM output; VENT_GND_CTRL output; VENT_PACE_CTRL output; Z_ATR_CTRL output; Z_VENT_CTRL output; FRONTEND_CTRL output; ATR_CMP_REF_PWM output; VENT_CMP_REF_PWM output
